simulink model "Fusion_Frame_Model_Architecture"  (R2018a)
settings: Solver=FixedStepAuto  StartTime=0.0  StopTime=SimulationTime  FixedStep=SamplingTime  RelTol=1e-3
undefined symbols (not defined in the file or in its folder): ACTIVATE_CAM, ACTIVATE_RAD, CAM1_detTimeStamp, CAM1_MeasNoise, CAM1_objClassID, CAM1_PX, CAM1_PY, CAM1_VX, CAM1_VY, CAM2_detTimeStamp, CAM2_MeasNoise, CAM2_objClassID, CAM2_PX, CAM2_PY, CAM2_VX, CAM2_VY, CAM3_detTimeStamp, CAM3_MeasNoise, CAM3_objClassID, CAM3_PX, CAM3_PY, CAM3_VX, CAM3_VY, CAM4_detTimeStamp, CAM4_MeasNoise, CAM4_objClassID, CAM4_PX, CAM4_PY, CAM4_VX, CAM4_VY, CAM5_detTimeStamp, CAM5_MeasNoise, CAM5_objClassID, CAM5_PX, CAM5_PY, CAM5_VX, CAM5_VY, CAM6_detTimeStamp, CAM6_MeasNoise, CAM6_objClassID, CAM6_PX, CAM6_PY, CAM6_VX, CAM6_VY, CAM7_detTimeStamp, CAM7_MeasNoise, CAM7_objClassID, CAM7_PX, CAM7_PY, CAM7_VX, CAM7_VY, CAM8_detTimeStamp, CAM8_MeasNoise, CAM8_objClassID, CAM8_PX, CAM8_PY, CAM8_VX, CAM8_VY, CAM_nMeas, CAM_TYPE ... (+181)
libraries: simulink_extras x4
(part 2 of 11)

== system Fusion_Frame_Model_Architecture/SENSOR_FUSION_SYSTEM/OBJECT_TRACKER_SENSOR_FUSION/RADAR_HOMOGENEOUS_FUSION/GATING ==
  MEAS : Inport
  RAD_PARAM : Inport  Port=2
  RADAR_CLUSTERS : Inport  Port=3
  TrackParamPred : Inport  Port=4
  FIND_UNASSOCIATED_CLUSTERS : Subsystem
  GET_DATA : Subsystem
  MEASUREMENT_TO_TRACK_GATING_AND_LOGLIKELIHOOD_COMPUTATION : Subsystem
  RESOLVE_GATING_AMBIGUITY : Subsystem
  GatedMeasFlag : Outport
  GatedMeasLogLikelihood : Outport  Port=2
  UnGatedMeasCluster : Outport  Port=3
  wires:
  MEAS/1 -> MEASUREMENT_TO_TRACK_GATING_AND_LOGLIKELIHOOD_COMPUTATION/4(Meas), FIND_UNASSOCIATED_CLUSTERS/3(measCLUSTERS)
  MEASUREMENT_TO_TRACK_GATING_AND_LOGLIKELIHOOD_COMPUTATION/2(GatedMeasFlagArray) -> RESOLVE_GATING_AMBIGUITY/3(GatedMeasFlagArrayIn)
  MEASUREMENT_TO_TRACK_GATING_AND_LOGLIKELIHOOD_COMPUTATION/3(GatedMeasLogLikelihood) -> RESOLVE_GATING_AMBIGUITY/4(GatedMeasLogLikelihoodIn)
  TrackParamPred/1 -> GET_DATA/1(TRACKS)
  GET_DATA/1(nTracksPred) -> MEASUREMENT_TO_TRACK_GATING_AND_LOGLIKELIHOOD_COMPUTATION/1(nTracks), RESOLVE_GATING_AMBIGUITY/1(nTracks)
  GET_DATA/2(TrackParam) -> MEASUREMENT_TO_TRACK_GATING_AND_LOGLIKELIHOOD_COMPUTATION/2(TrackParamPred)
  MEASUREMENT_TO_TRACK_GATING_AND_LOGLIKELIHOOD_COMPUTATION/1(nMeas) -> RESOLVE_GATING_AMBIGUITY/2(nMeas)
  RESOLVE_GATING_AMBIGUITY/1(GatedMeasFlagArray) -> GatedMeasFlag/1, FIND_UNASSOCIATED_CLUSTERS/1(GatedMeasFlagArray)
  RADAR_CLUSTERS/1 -> FIND_UNASSOCIATED_CLUSTERS/2(Clusters)
  RESOLVE_GATING_AMBIGUITY/2(GatedMeasLogLikelihood) -> GatedMeasLogLikelihood/1
  FIND_UNASSOCIATED_CLUSTERS/1(UngatedCLUSTERS) -> UnGatedMeasCluster/1
  RAD_PARAM/1 -> MEASUREMENT_TO_TRACK_GATING_AND_LOGLIKELIHOOD_COMPUTATION/3(SnsrParam)

== system Fusion_Frame_Model_Architecture/SENSOR_FUSION_SYSTEM/OBJECT_TRACKER_SENSOR_FUSION/RADAR_HOMOGENEOUS_FUSION/SEGREGATE_CLUSTER ==
  RADAR_MEAS : Inport
  RADAR_CLUSTERS : Inport  Port=2
  Bus Creator : BusCreator  Inputs=5  OutDataTypeStr=Bus: RAD_MEAS_MAT_CTS  NonVirtualBus=on
      settings: InheritFromInputs=off
  MATLAB Function : MATLAB Function  TreatAsAtomicUnit=on
  Spatially_Alligned_Snsr_Meas_Plots : Subsystem
  RADAR_CLSTR_MEAS : Outport
  wires:
  RADAR_MEAS/1 -> MATLAB Function/1(SENSORMeasCTS)
  RADAR_CLUSTERS/1 -> MATLAB Function/2(SENSOR_CLUSTERS)
  Bus Creator/1 -> Spatially_Alligned_Snsr_Meas_Plots/1(RAD_MEAS), RADAR_CLSTR_MEAS/1
  MATLAB Function/1(MeasArray) -> Bus Creator/1  "MeasArray"
  MATLAB Function/2(MeasCovariance) -> Bus Creator/2  "MeasCovariance"
  MATLAB Function/3(ClusterRef) -> Bus Creator/3  "MeasRef"
  MATLAB Function/4(ValidMeasCount) -> Bus Creator/4  "ValidMeasCount"
  MATLAB Function/5(ValidCumulativeMeasCount) -> Bus Creator/5  "ValidCumulativeMeasCount"

== system Fusion_Frame_Model_Architecture/SENSOR_FUSION_SYSTEM/OBJECT_TRACKER_SENSOR_FUSION/RADAR_HOMOGENEOUS_FUSION/SIMPLYFIED_DBSCAN_FOR_RADAR_MEASUREMENT_GROUPING ==
  RADAR_MEAS : Inport
  DBSCAN_MEASUREMENT_GROUPING : Subsystem  TreatAsAtomicUnit=on
  GET_NUM_OF_MEAS : Subsystem
  RADAR_CLUSTERS : Outport
  wires:
  GET_NUM_OF_MEAS/1(nMeas) -> DBSCAN_MEASUREMENT_GROUPING/1(nMeas)
  RADAR_MEAS/1 -> GET_NUM_OF_MEAS/1(RAD_MEAS_CTS), DBSCAN_MEASUREMENT_GROUPING/2(Meas)
  DBSCAN_MEASUREMENT_GROUPING/1(RADAR_CLUSTERS) -> RADAR_CLUSTERS/1

== system Fusion_Frame_Model_Architecture/SENSOR_FUSION_SYSTEM/OBJECT_TRACKER_SENSOR_FUSION/RADAR_HOMOGENEOUS_FUSION/STATE_PREDICTION ==
  TrackParamPrev : Inport
  GET_DATA : Subsystem
  SET_DATA : Subsystem
  TRACK_STATE_PREDICTION : Subsystem
  Unit Delay : UnitDelay  InitialCondition=TRACK_EST_RAD_INIT  SampleTime=-1
  TrackParamPred : Outport
  wires:
  TrackParamPrev/1 -> Unit Delay/1
  Unit Delay/1 -> GET_DATA/1(TRACKS), SET_DATA/1(TRACKS_in)
  GET_DATA/1(nTracksPrev) -> TRACK_STATE_PREDICTION/1(nTracks)
  GET_DATA/2(TrackParam) -> TRACK_STATE_PREDICTION/2(TrackParamPred)
  TRACK_STATE_PREDICTION/1(StatePredBus) -> SET_DATA/2(TrackParam)
  SET_DATA/1(TRACKS) -> TrackParamPred/1

== system Fusion_Frame_Model_Architecture/SENSOR_FUSION_SYSTEM/OBJECT_TRACKER_SENSOR_FUSION/RADAR_HOMOGENEOUS_FUSION/TRACK_MANAGER ==
  TrackParamIn : Inport
  UnGatedClusters : Inport  Port=2
  Grid : Inport  Port=3
  Bus Creator : BusCreator  Inputs=6  OutDataTypeStr=Bus: TRACK_ESTIMATES_BUS  NonVirtualBus=on
      settings: InheritFromInputs=off
  Bus Selector : BusSelector  OutputSignals=nValidTracks,TrackParam,TrackIDList,IsTrackIDused,FirstAvailableIDindex,LastAvailableIDindex
  Terminator : Terminator
  Terminator1 : Terminator
  TrackParamUpd : Outport
  wires:
  UnGatedClusters/1 -> Terminator/1
  Bus Creator/1 -> TrackParamUpd/1
  Bus Selector/4 -> Bus Creator/4  "<IsTrackIDused>"
  Bus Selector/2 -> Bus Creator/2  "<TrackParam>"
  Bus Selector/3 -> Bus Creator/3  "<TrackIDList>"
  TrackParamIn/1 -> Bus Selector/1
  Bus Selector/1 -> Bus Creator/1  "<nValidTracks>"
  Bus Selector/5 -> Bus Creator/5  "<FirstAvailableIDindex>"
  Bus Selector/6 -> Bus Creator/6  "<LastAvailableIDindex>"
  Grid/1 -> Terminator1/1

== system Fusion_Frame_Model_Architecture/SENSOR_FUSION_SYSTEM/OBJECT_TRACKER_SENSOR_FUSION/SENSOR_LAYOUT_AND_CHRACTERIZATION/PRE_COMPUTE_SENSOR_FOV_GRID ==
  RADSnsrParam : Inport
  CAMSnsrParam : Inport  Port=2
  COMPUTE_CAMERA_SNSR_GRID : Subsystem
  COMPUTE_GRID_DIMENSION : Subsystem
  COMPUTE_RADAR_SNSR_GRID : Subsystem
  CREATE_GRID : Subsystem  TreatAsAtomicUnit=on
  SET_DATA : Subsystem
  GRID_CHARACTERIZATION : Outport
  wires:
  RADSnsrParam/1 -> COMPUTE_RADAR_SNSR_GRID/1(SnsrParam)
  COMPUTE_GRID_DIMENSION/2(Cy) -> CREATE_GRID/2(Cy)
  COMPUTE_GRID_DIMENSION/3(GridParam) -> [GridParam], CREATE_GRID/3(GridParam)
  COMPUTE_GRID_DIMENSION/1(Cx) -> CREATE_GRID/1(Cx)
  CREATE_GRID/1(CellIDVectorUpd) -> COMPUTE_CAMERA_SNSR_GRID/1(GridIDVector), COMPUTE_RADAR_SNSR_GRID/3(GridIDVector)
  [GridParam] -> COMPUTE_RADAR_SNSR_GRID/2(GridParam)
  [GridParam] -> COMPUTE_CAMERA_SNSR_GRID/2(GridParam)
  CAMSnsrParam/1 -> COMPUTE_CAMERA_SNSR_GRID/3(SnsrParam)
  [GridParam] -> SET_DATA/1(GRID_PARAM)  "GRID_PARAM"
  COMPUTE_RADAR_SNSR_GRID/1(RegionConfidence) -> SET_DATA/2(RAD_REGION_CONFIDENCE)  "RAD_REGION_CONFIDENCE"
  COMPUTE_RADAR_SNSR_GRID/2(FOVOverlap) -> SET_DATA/3(RAD_FOV_OVERLAP)  "RAD_FOV_OVERLAP"
  COMPUTE_CAMERA_SNSR_GRID/1(RegionConfidence) -> SET_DATA/4(CAM_REGION_CONFIDENCE)  "CAM_REGION_CONFIDENCE"
  COMPUTE_CAMERA_SNSR_GRID/2(FOVOverlap) -> SET_DATA/5(CAM_FOV_OVERLAP)  "CAM_FOV_OVERLAP"
  SET_DATA/1(GRID_CHARACTERIZATION) -> GRID_CHARACTERIZATION/1

== system Fusion_Frame_Model_Architecture/SENSOR_FUSION_SYSTEM/OBJECT_TRACKER_SENSOR_FUSION/SENSOR_LAYOUT_AND_CHRACTERIZATION/SET_SENSOR_CALLIBRATION_PARAMETER ==
  CamCalibParam : Inport  OutDataTypeStr=Bus: CAM_SENSOR_PARAM  PortDimensions=nCameraActive  BusOutputAsStruct=on
  RADSnsrParam : Inport  Port=2  OutDataTypeStr=Bus: RAD_SENSOR_PARAM  PortDimensions=1
  SET_CAMERA_SENSOR_PARAM : Subsystem  TreatAsAtomicUnit=on
  SET_RADAR_SENSOR_PARAM : Subsystem
  RadarCalibParamUpd : Outport
  CameraCalibParamUpd : Outport  Port=2
  wires:
  SET_CAMERA_SENSOR_PARAM/1(CAMSnsrParamUpd) -> CameraCalibParamUpd/1
  CamCalibParam/1 -> SET_CAMERA_SENSOR_PARAM/1(CAMSnsrParam)
  RADSnsrParam/1 -> SET_RADAR_SENSOR_PARAM/1(RADSnsrParam)
  SET_RADAR_SENSOR_PARAM/1(RADSnsrParamUpd) -> RadarCalibParamUpd/1

== system Fusion_Frame_Model_Architecture/SENSOR_FUSION_SYSTEM/OBJECT_TRACKER_SENSOR_FUSION/SPATIAL_ALLIGNMENT1/CAMERA_MEASUREMENTS_SPATIAL_ALLIGNMENT ==
  CameraCalibParam : Inport  BusOutputAsStruct=on
  C1 : Inport  Port=2
  C2 : Inport  Port=3
  C3 : Inport  Port=4
  C4 : Inport  Port=5
  C5 : Inport  Port=6
  C6 : Inport  Port=7
  C7 : Inport  Port=8
  C8 : Inport  Port=9
  For Iterator Subsystem : Subsystem  TreatAsAtomicUnit=on
  RadarMeasurementIndexes2 : Subsystem
  StartingIndexes1 : Subsystem
  CameraMeasTransformed : Outport
  wires:
  CameraCalibParam/1 -> For Iterator Subsystem/1(CameraCallibrationParam), StartingIndexes1/1(SnsrCallib)
  C6/1 -> For Iterator Subsystem/8(C6)
  C3/1 -> For Iterator Subsystem/5(C3)
  C4/1 -> For Iterator Subsystem/6(C4)
  C2/1 -> For Iterator Subsystem/4(C2)
  C1/1 -> For Iterator Subsystem/3(C1)
  StartingIndexes1/1(StartingIndexes) -> For Iterator Subsystem/2(RadarStartingIdx)
  C5/1 -> For Iterator Subsystem/7(C5)
  C7/1 -> For Iterator Subsystem/9(C7)
  C8/1 -> For Iterator Subsystem/10(C8)
  For Iterator Subsystem/2(CameraMeasTransformed) -> RadarMeasurementIndexes2/2(CTSmeasMAT)
  RadarMeasurementIndexes2/1(CTSmeasMATout) -> CameraMeasTransformed/1
  For Iterator Subsystem/4(CameraMeasRef) -> RadarMeasurementIndexes2/4(CTSRefMAT)
  For Iterator Subsystem/3(CameraMeasCOVTransformed) -> RadarMeasurementIndexes2/3(CTSCovMAT)
  For Iterator Subsystem/1(MaxNoValidMeas) -> RadarMeasurementIndexes2/1(validMeasCount)

== system Fusion_Frame_Model_Architecture/SENSOR_FUSION_SYSTEM/OBJECT_TRACKER_SENSOR_FUSION/SPATIAL_ALLIGNMENT1/GET_CAM_MEAS ==
  CameraParam : Inport
  CameraMeas : Inport  Port=2
  Bus Selector1 : BusSelector  OutputSignals=C1,C2,C3,C4,C5,C6,C7,C8
  Bus Selector2 : BusSelector  OutputSignals=CameraExtrinsics
  SnsrParam : Outport
  <C1> : Outport  Port=2
  <C2> : Outport  Port=3
  <C3> : Outport  Port=4
  <C4> : Outport  Port=5
  <C5> : Outport  Port=6
  <C6> : Outport  Port=7
  <C7> : Outport  Port=8
  <C8> : Outport  Port=9
  wires:
  Bus Selector1/4 -> <C4>/1  "<C4>"
  Bus Selector1/6 -> <C6>/1  "<C6>"
  Bus Selector1/5 -> <C5>/1  "<C5>"
  CameraMeas/1 -> Bus Selector1/1
  Bus Selector1/1 -> <C1>/1  "<C1>"
  Bus Selector1/7 -> <C7>/1  "<C7>"
  Bus Selector1/8 -> <C8>/1  "<C8>"
  Bus Selector1/2 -> <C2>/1  "<C2>"
  Bus Selector1/3 -> <C3>/1  "<C3>"
  CameraParam/1 -> Bus Selector2/1
  Bus Selector2/1 -> SnsrParam/1  "<CameraExtrinsics>"

== system Fusion_Frame_Model_Architecture/SENSOR_FUSION_SYSTEM/OBJECT_TRACKER_SENSOR_FUSION/SPATIAL_ALLIGNMENT1/GET_RAD_MEAS ==
  RadarParam : Inport
  RadarMeas : Inport  Port=2
  Bus Selector : BusSelector  OutputSignals=R1,R2,R3,R4,R5,R6
  Bus Selector1 : BusSelector  OutputSignals=RadarExtrinsics
  SnsrParam : Outport
  <R1> : Outport  Port=2
  <R2> : Outport  Port=3
  <R3> : Outport  Port=4
  <R4> : Outport  Port=5
  <R5> : Outport  Port=6
  <R6> : Outport  Port=7
  wires:
  Bus Selector/1 -> <R1>/1  "<R1>"
  Bus Selector/2 -> <R2>/1  "<R2>"
  Bus Selector/3 -> <R3>/1  "<R3>"
  Bus Selector/6 -> <R6>/1  "<R6>"
  Bus Selector/4 -> <R4>/1  "<R4>"
  Bus Selector/5 -> <R5>/1  "<R5>"
  RadarMeas/1 -> Bus Selector/1
  Bus Selector1/1 -> SnsrParam/1  "<RadarExtrinsics>"
  RadarParam/1 -> Bus Selector1/1

== system Fusion_Frame_Model_Architecture/SENSOR_FUSION_SYSTEM/OBJECT_TRACKER_SENSOR_FUSION/SPATIAL_ALLIGNMENT1/RADAR_MEASUREMENTS_SPATIAL_ALLIGNMENT ==
  RadarCalibParam : Inport  BusOutputAsStruct=on
  R1 : Inport  Port=2
  R2 : Inport  Port=3
  R3 : Inport  Port=4
  R4 : Inport  Port=5
  R5 : Inport  Port=6
  R6 : Inport  Port=7
  RADAR_MEASUREMENTS_SPATIAL_ALLIGNMENT : Subsystem  TreatAsAtomicUnit=on
  SET_MEASUREMENTS : Subsystem
  StartingIndexes1 : Subsystem
  RadarMeasTransformed : Outport
  wires:
  StartingIndexes1/1(StartingIndexes) -> RADAR_MEASUREMENTS_SPATIAL_ALLIGNMENT/2(RadarStartingIdx)
  R1/1 -> RADAR_MEASUREMENTS_SPATIAL_ALLIGNMENT/3(R1)
  R2/1 -> RADAR_MEASUREMENTS_SPATIAL_ALLIGNMENT/4(R2)
  R4/1 -> RADAR_MEASUREMENTS_SPATIAL_ALLIGNMENT/6(R4)
  R5/1 -> RADAR_MEASUREMENTS_SPATIAL_ALLIGNMENT/7(R5)
  RadarCalibParam/1 -> RADAR_MEASUREMENTS_SPATIAL_ALLIGNMENT/1(RadarCallibrationParam), StartingIndexes1/1(SnsrCallib)
  R6/1 -> RADAR_MEASUREMENTS_SPATIAL_ALLIGNMENT/8(R6)
  R3/1 -> RADAR_MEASUREMENTS_SPATIAL_ALLIGNMENT/5(R3)
  RADAR_MEASUREMENTS_SPATIAL_ALLIGNMENT/1(RadarMeasTransformed) -> SET_MEASUREMENTS/1(CTSmeasMAT)
  RADAR_MEASUREMENTS_SPATIAL_ALLIGNMENT/4(MaxNoValidMeas) -> SET_MEASUREMENTS/4(validMeasCount)
  SET_MEASUREMENTS/1(CTSmeasMATout) -> RadarMeasTransformed/1
  RADAR_MEASUREMENTS_SPATIAL_ALLIGNMENT/2(RadarMeasCOVTransformed) -> SET_MEASUREMENTS/2(CTSCovMAT)
  RADAR_MEASUREMENTS_SPATIAL_ALLIGNMENT/3(RadarMeasRef) -> SET_MEASUREMENTS/3(CTSRefMAT)

== system Fusion_Frame_Model_Architecture/SENSOR_FUSION_SYSTEM/OBJECT_TRACKER_SENSOR_FUSION/TRACKS_TRAJECTORY_COMPUTATION/EGO_COMPENSATE_TRAJECTORY_HISTORY_BUFFER ==
  RAD_CAM_TRACKS_FUS : Inport
  TRAJECTORIES : Inport  Port=2
  Bus Creator : BusCreator  Inputs=2  OutDataTypeStr=Bus: TRAJECTORY_HISTORY_BUS  NonVirtualBus=on
      settings: InheritFromInputs=off
  Bus Selector : BusSelector  OutputSignals=nConfirmedTracks,TrackHistory
  Terminator : Terminator
  TRAJECTORIES_UPD : Outport
  wires:
  RAD_CAM_TRACKS_FUS/1 -> Terminator/1
  Bus Selector/2 -> Bus Creator/2  "<TrackHistory>"
  Bus Selector/1 -> Bus Creator/1  "<nConfirmedTracks>"
  TRAJECTORIES/1 -> Bus Selector/1
  Bus Creator/1 -> TRAJECTORIES_UPD/1

== system Fusion_Frame_Model_Architecture/SENSOR_FUSION_SYSTEM/OBJECT_TRACKER_SENSOR_FUSION/TRACKS_TRAJECTORY_COMPUTATION/UPDATE_TRAJECTORY_BUFFER_WITH_CURRENT_TRACK_DATA ==
  RAD_CAM_TRACKS_FUS : Inport
  TRAJECTORIES : Inport  Port=2
  Terminator : Terminator
  Unit Delay : UnitDelay  InitialCondition=TRACK_HISTORY_INIT  SampleTime=-1
  TRAJECTORIES_UPD : Outport
  wires:
  TRAJECTORIES/1 -> Unit Delay/1
  Unit Delay/1 -> TRAJECTORIES_UPD/1
  RAD_CAM_TRACKS_FUS/1 -> Terminator/1

== system Fusion_Frame_Model_Architecture/SENSOR_FUSION_SYSTEM/ROAD_GEOMETRY_CAMERA_FUSION/EGO_LANE_CENTER_LINE_ESTIMATION_FROM_LEFT_BOUNDARY/CURVE_FITTING_BY_LEAST_SQUARES ==
  Points : Inport
  Ground : Ground
  Terminator : Terminator
  PolynomialCoefficients : Outport
  wires:
  Points/1 -> Terminator/1
  Ground/1 -> PolynomialCoefficients/1

== system Fusion_Frame_Model_Architecture/SENSOR_FUSION_SYSTEM/ROAD_GEOMETRY_CAMERA_FUSION/EGO_LANE_CENTER_LINE_ESTIMATION_FROM_LEFT_BOUNDARY/GENERATE_POINTS_AT_EGO_LANE_CENTER ==
  PointsAlongTheLine : Inport
  EgoLaneWidth : Inport  Port=2
  Ground : Ground
  Terminator : Terminator
  Terminator1 : Terminator
  PointsAlongEgoLaneCenter : Outport
  wires:
  PointsAlongTheLine/1 -> Terminator/1
  Ground/1 -> PointsAlongEgoLaneCenter/1
  EgoLaneWidth/1 -> Terminator1/1

== system Fusion_Frame_Model_Architecture/SENSOR_FUSION_SYSTEM/ROAD_GEOMETRY_CAMERA_FUSION/EGO_LANE_CENTER_LINE_ESTIMATION_FROM_LEFT_BOUNDARY/INTERPOLATE_POINTS_ALONG_THE_LINE ==
  LEFT_LINE_TRACK : Inport
  Ground : Ground
  Terminator : Terminator
  PointsAlongTheLine : Outport
  wires:
  LEFT_LINE_TRACK/1 -> Terminator/1
  Ground/1 -> PointsAlongTheLine/1

== system Fusion_Frame_Model_Architecture/SENSOR_FUSION_SYSTEM/ROAD_GEOMETRY_CAMERA_FUSION/EGO_LANE_CENTER_LINE_ESTIMATION_FROM_LEFT_BOUNDARY/KALMAN_FILTER_STATE_UPDATE ==
  CenterLineHypothesis : Inport
  CenterLinePred : Inport  Port=2
  Terminator : Terminator
  Unit Delay : UnitDelay  InitialCondition=LANE_LINE_TRACK  SampleTime=-1
  CenterLineHypUpd : Outport
  wires:
  CenterLineHypothesis/1 -> Terminator/1
  CenterLinePred/1 -> Unit Delay/1
  Unit Delay/1 -> CenterLineHypUpd/1

== system Fusion_Frame_Model_Architecture/SENSOR_FUSION_SYSTEM/ROAD_GEOMETRY_CAMERA_FUSION/EGO_LANE_CENTER_LINE_ESTIMATION_FROM_LEFT_BOUNDARY/POLYNOMIAL_TO_CLOTHOID_CONVERSION ==
  PolynomialCoefficients : Inport
  Ground : Ground
  Terminator : Terminator
  ClothoidCoefficients : Outport
  wires:
  PolynomialCoefficients/1 -> Terminator/1
  Ground/1 -> ClothoidCoefficients/1

== system Fusion_Frame_Model_Architecture/SENSOR_FUSION_SYSTEM/ROAD_GEOMETRY_CAMERA_FUSION/EGO_LANE_CENTER_LINE_ESTIMATION_FROM_RIGHT_BOUNDARY/CURVE_FITTING_BY_LEAST_SQUARES ==
  Points : Inport
  Ground : Ground
  Terminator : Terminator
  PolynomialCoefficients : Outport
  wires:
  Points/1 -> Terminator/1
  Ground/1 -> PolynomialCoefficients/1

== system Fusion_Frame_Model_Architecture/SENSOR_FUSION_SYSTEM/ROAD_GEOMETRY_CAMERA_FUSION/EGO_LANE_CENTER_LINE_ESTIMATION_FROM_RIGHT_BOUNDARY/GENERATE_POINTS_AT_EGO_LANE_CENTER ==
  PointsAlongTheLine : Inport
  EgoLaneWidth : Inport  Port=2
  Ground : Ground
  Terminator : Terminator
  Terminator1 : Terminator
  PointsAlongEgoLaneCenter : Outport
  wires:
  PointsAlongTheLine/1 -> Terminator/1
  Ground/1 -> PointsAlongEgoLaneCenter/1
  EgoLaneWidth/1 -> Terminator1/1

== system Fusion_Frame_Model_Architecture/SENSOR_FUSION_SYSTEM/ROAD_GEOMETRY_CAMERA_FUSION/EGO_LANE_CENTER_LINE_ESTIMATION_FROM_RIGHT_BOUNDARY/INTERPOLATE_POINTS_ALONG_THE_LINE ==
  LEFT_LINE_TRACK : Inport
  Ground : Ground
  Terminator : Terminator
  PointsAlongTheLine : Outport
  wires:
  LEFT_LINE_TRACK/1 -> Terminator/1
  Ground/1 -> PointsAlongTheLine/1

== system Fusion_Frame_Model_Architecture/SENSOR_FUSION_SYSTEM/ROAD_GEOMETRY_CAMERA_FUSION/EGO_LANE_CENTER_LINE_ESTIMATION_FROM_RIGHT_BOUNDARY/KALMAN_FILTER_STATE_UPDATE ==
  CenterLineHypothesis : Inport
  CenterLinePred : Inport  Port=2
  Terminator : Terminator
  Unit Delay : UnitDelay  InitialCondition=LANE_LINE_TRACK  SampleTime=-1
  CenterLineHypUpd : Outport
  wires:
  CenterLineHypothesis/1 -> Terminator/1
  CenterLinePred/1 -> Unit Delay/1
  Unit Delay/1 -> CenterLineHypUpd/1

== system Fusion_Frame_Model_Architecture/SENSOR_FUSION_SYSTEM/ROAD_GEOMETRY_CAMERA_FUSION/EGO_LANE_CENTER_LINE_ESTIMATION_FROM_RIGHT_BOUNDARY/POLYNOMIAL_TO_CLOTHOID_CONVERSION ==
  PolynomialCoefficients : Inport
  Ground : Ground
  Terminator : Terminator
  ClothoidCoefficients : Outport
  wires:
  PolynomialCoefficients/1 -> Terminator/1
  Ground/1 -> ClothoidCoefficients/1

== system Fusion_Frame_Model_Architecture/SENSOR_FUSION_SYSTEM/ROAD_GEOMETRY_CAMERA_FUSION/EGO_LANE_CENTER_LINE_HYPOTHESIS_FUSION/EGO_LANE_CENTER_LINE_PREDICTION ==
  EGO_LANE_CENTER_LINE : Inport
  Bus Creator : BusCreator  Inputs=7  OutDataTypeStr=Bus: ClothoidParamBus  NonVirtualBus=on
      settings: InheritFromInputs=off
  Bus Selector : BusSelector  OutputSignals=LateralOffset,HeadingAngle,Curvature,CurvatureDerivative,CurveLengthStart,CurveLength,ErrCOV
  EGO_LANE_CENTER_LINE_PRED : Outport
  wires:
  Bus Creator/1 -> EGO_LANE_CENTER_LINE_PRED/1
  Bus Selector/6 -> Bus Creator/6  "<CurveLength>"
  Bus Selector/5 -> Bus Creator/5  "<CurveLengthStart>"
  Bus Selector/4 -> Bus Creator/4  "<CurvatureDerivative>"
  Bus Selector/1 -> Bus Creator/1  "<LateralOffset>"
  Bus Selector/3 -> Bus Creator/3  "<Curvature>"
  EGO_LANE_CENTER_LINE/1 -> Bus Selector/1
  Bus Selector/2 -> Bus Creator/2  "<HeadingAngle>"
  Bus Selector/7 -> Bus Creator/7  "<ErrCOV>"

== system Fusion_Frame_Model_Architecture/SENSOR_FUSION_SYSTEM/ROAD_GEOMETRY_CAMERA_FUSION/EGO_LANE_CENTER_LINE_HYPOTHESIS_FUSION/HYPOTHESIS_MERGE ==
  EGO_LANE_CENTER_LINE_HYP1 : Inport
  weight : Inport  Port=2
  EGO_LANE_CENTER_LINE_HYP2 : Inport  Port=3
  Terminator1 : Terminator
  Terminator2 : Terminator
  EGO_LANE_CENTER_LINE : Outport
  wires:
  EGO_LANE_CENTER_LINE_HYP1/1 -> EGO_LANE_CENTER_LINE/1
  EGO_LANE_CENTER_LINE_HYP2/1 -> Terminator1/1
  weight/1 -> Terminator2/1

== system Fusion_Frame_Model_Architecture/SENSOR_FUSION_SYSTEM/ROAD_GEOMETRY_CAMERA_FUSION/EGO_LANE_CENTER_LINE_HYPOTHESIS_FUSION/WEIGHTAGE_COMPUTATION ==
  EGO_LANE_CENTER_LINE_HYP1 : Inport
  EGO_LANE_CENTER_LINE_HYP2 : Inport  Port=2
  Ground : Ground
  Terminator : Terminator
  Terminator1 : Terminator
  weight : Outport
  wires:
  EGO_LANE_CENTER_LINE_HYP1/1 -> Terminator/1
  EGO_LANE_CENTER_LINE_HYP2/1 -> Terminator1/1
  Ground/1 -> weight/1

== system Fusion_Frame_Model_Architecture/SENSOR_FUSION_SYSTEM/ROAD_GEOMETRY_CAMERA_FUSION/EGO_LANE_LEFT_BOUNDARY_LINE_FUSION/FIND_UNGATED_LINE_MEASUREMENTS ==
  GatedMeasIndex : Inport
  EGO_LANE_LEFT_LINE_MEAS : Inport  Port=2
  Ground : Ground
  Terminator1 : Terminator
  Terminator2 : Terminator
  UnGatedMeasIndex : Outport
  wires:
  EGO_LANE_LEFT_LINE_MEAS/1 -> Terminator1/1
  GatedMeasIndex/1 -> Terminator2/1
  Ground/1 -> UnGatedMeasIndex/1

== system Fusion_Frame_Model_Architecture/SENSOR_FUSION_SYSTEM/ROAD_GEOMETRY_CAMERA_FUSION/EGO_LANE_LEFT_BOUNDARY_LINE_FUSION/LANE_LINE_MEASUREMENT_TO_TRACK_FUSION ==
  GatedMeasIndex : Inport
  TrackParamPred : Inport  Port=2
  EGO_LANE_LEFT_LINE_MEAS : Inport  Port=3
  Terminator1 : Terminator
  Terminator2 : Terminator
  TrackParamUpd : Outport
  wires:
  TrackParamPred/1 -> TrackParamUpd/1
  EGO_LANE_LEFT_LINE_MEAS/1 -> Terminator1/1
  GatedMeasIndex/1 -> Terminator2/1

== system Fusion_Frame_Model_Architecture/SENSOR_FUSION_SYSTEM/ROAD_GEOMETRY_CAMERA_FUSION/EGO_LANE_LEFT_BOUNDARY_LINE_FUSION/LANE_LINE_MEASUREMENT_TO_TRACK_GATING ==
  TrackParamPred : Inport
  EGO_LANE_LEFT_LINE_MEAS : Inport  Port=2
  Ground : Ground
  Terminator : Terminator
  Terminator1 : Terminator
  GatedMeasIndex : Outport
  wires:
  TrackParamPred/1 -> Terminator/1
  Ground/1 -> GatedMeasIndex/1
  EGO_LANE_LEFT_LINE_MEAS/1 -> Terminator1/1

== system Fusion_Frame_Model_Architecture/SENSOR_FUSION_SYSTEM/ROAD_GEOMETRY_CAMERA_FUSION/EGO_LANE_LEFT_BOUNDARY_LINE_FUSION/LANE_LINE_STATE_PREDICTION ==
  TrackParamPrev : Inport
  Unit Delay : UnitDelay  InitialCondition=LANE_LINE_TRACK  SampleTime=-1
  TrackParamPred : Outport
  wires:
  TrackParamPrev/1 -> Unit Delay/1
  Unit Delay/1 -> TrackParamPred/1

== system Fusion_Frame_Model_Architecture/SENSOR_FUSION_SYSTEM/ROAD_GEOMETRY_CAMERA_FUSION/EGO_LANE_LEFT_BOUNDARY_LINE_FUSION/LINE_TRACK_MANAGER ==
  UnGatedMeasIndex : Inport
  TrackParamUpd_in : Inport  Port=2
  Line_Measurements : Inport  Port=3
  Bus Creator : BusCreator  Inputs=7  OutDataTypeStr=Bus: ClothoidParamBus  NonVirtualBus=on
      settings: InheritFromInputs=off
  Bus Selector : BusSelector  OutputSignals=LateralOffset,HeadingAngle,Curvature,CurvatureDerivative,CurveLengthStart,CurveLength,ErrCOV
  Terminator : Terminator
  Terminator1 : Terminator
  TrackParamUpd : Outport
  wires:
  UnGatedMeasIndex/1 -> Terminator/1
  Line_Measurements/1 -> Terminator1/1
  Bus Selector/7 -> Bus Creator/7  "<ErrCOV>"
  Bus Selector/3 -> Bus Creator/3  "<Curvature>"
  Bus Creator/1 -> TrackParamUpd/1
  Bus Selector/4 -> Bus Creator/4  "<CurvatureDerivative>"
  Bus Selector/6 -> Bus Creator/6  "<CurveLength>"
  Bus Selector/1 -> Bus Creator/1  "<LateralOffset>"
  Bus Selector/2 -> Bus Creator/2  "<HeadingAngle>"
  Bus Selector/5 -> Bus Creator/5  "<CurveLengthStart>"
  TrackParamUpd_in/1 -> Bus Selector/1

== system Fusion_Frame_Model_Architecture/SENSOR_FUSION_SYSTEM/ROAD_GEOMETRY_CAMERA_FUSION/EGO_LANE_RIGHT_BOUNDARY_LINE_FUSION/FIND_UNGATED_LINE_MEASUREMENTS ==
  GatedMeasIndex : Inport
  EGO_LANE_RIGHT_LINE_MEAS : Inport  Port=2
  Ground : Ground
  Terminator1 : Terminator
  Terminator2 : Terminator
  UnGatedMeasIndex : Outport
  wires:
  EGO_LANE_RIGHT_LINE_MEAS/1 -> Terminator1/1
  GatedMeasIndex/1 -> Terminator2/1
  Ground/1 -> UnGatedMeasIndex/1

== system Fusion_Frame_Model_Architecture/SENSOR_FUSION_SYSTEM/ROAD_GEOMETRY_CAMERA_FUSION/EGO_LANE_RIGHT_BOUNDARY_LINE_FUSION/LANE_LINE_MEASUREMENT_TO_TRACK_FUSION ==
  GatedMeasIndex : Inport
  TrackParamPred : Inport  Port=2
  EGO_LANE_RIGHT_LINE_MEAS : Inport  Port=3
  Terminator1 : Terminator
  Terminator2 : Terminator
  TrackParamUpd : Outport
  wires:
  TrackParamPred/1 -> TrackParamUpd/1
  EGO_LANE_RIGHT_LINE_MEAS/1 -> Terminator1/1
  GatedMeasIndex/1 -> Terminator2/1

== system Fusion_Frame_Model_Architecture/SENSOR_FUSION_SYSTEM/ROAD_GEOMETRY_CAMERA_FUSION/EGO_LANE_RIGHT_BOUNDARY_LINE_FUSION/LANE_LINE_MEASUREMENT_TO_TRACK_GATING ==
  TrackParamPred : Inport
  EGO_LANE_RIGHT_LINE_MEAS : Inport  Port=2
  Ground : Ground
  Terminator : Terminator
  Terminator1 : Terminator
  GatedMeasIndex : Outport
  wires:
  TrackParamPred/1 -> Terminator/1
  Ground/1 -> GatedMeasIndex/1
  EGO_LANE_RIGHT_LINE_MEAS/1 -> Terminator1/1

== system Fusion_Frame_Model_Architecture/SENSOR_FUSION_SYSTEM/ROAD_GEOMETRY_CAMERA_FUSION/EGO_LANE_RIGHT_BOUNDARY_LINE_FUSION/LANE_LINE_STATE_PREDICTION ==
  TrackParamPrev : Inport
  Unit Delay : UnitDelay  InitialCondition=LANE_LINE_TRACK  SampleTime=-1
  TrackParamPred : Outport
  wires:
  TrackParamPrev/1 -> Unit Delay/1
  Unit Delay/1 -> TrackParamPred/1

== system Fusion_Frame_Model_Architecture/SENSOR_FUSION_SYSTEM/ROAD_GEOMETRY_CAMERA_FUSION/EGO_LANE_RIGHT_BOUNDARY_LINE_FUSION/LINE_TRACK_MANAGER ==
  UnGatedMeasIndex : Inport
  TrackParamUpd_in : Inport  Port=2
  Line_Measurements : Inport  Port=3
  Bus Creator : BusCreator  Inputs=7  OutDataTypeStr=Bus: ClothoidParamBus  NonVirtualBus=on
      settings: InheritFromInputs=off
  Bus Selector : BusSelector  OutputSignals=LateralOffset,HeadingAngle,Curvature,CurvatureDerivative,CurveLengthStart,CurveLength,ErrCOV
  Terminator : Terminator
  Terminator1 : Terminator
  TrackParamUpd : Outport
  wires:
  UnGatedMeasIndex/1 -> Terminator/1
  Line_Measurements/1 -> Terminator1/1
  Bus Selector/7 -> Bus Creator/7  "<ErrCOV>"
  Bus Selector/3 -> Bus Creator/3  "<Curvature>"
  Bus Creator/1 -> TrackParamUpd/1
  Bus Selector/4 -> Bus Creator/4  "<CurvatureDerivative>"
  Bus Selector/6 -> Bus Creator/6  "<CurveLength>"
  Bus Selector/1 -> Bus Creator/1  "<LateralOffset>"
  Bus Selector/2 -> Bus Creator/2  "<HeadingAngle>"
  Bus Selector/5 -> Bus Creator/5  "<CurveLengthStart>"
  TrackParamUpd_in/1 -> Bus Selector/1

== system Fusion_Frame_Model_Architecture/SENSOR_FUSION_SYSTEM/ROAD_GEOMETRY_CAMERA_FUSION/EGO_LANE_WIDTH_ESTIMATION/COMPUTE_SLOPE_AT_THE_POINTS ==
  SMALLER_CURVE : Inport
  POINTS : Inport  Port=2
  Ground : Ground
  Terminator : Terminator
  Terminator1 : Terminator
  SLOPE : Outport
  wires:
  SMALLER_CURVE/1 -> Terminator/1
  Ground/1 -> SLOPE/1
  POINTS/1 -> Terminator1/1

== system Fusion_Frame_Model_Architecture/SENSOR_FUSION_SYSTEM/ROAD_GEOMETRY_CAMERA_FUSION/EGO_LANE_WIDTH_ESTIMATION/COMPUTE_WIDTH_ALONG_THE_POINTS ==
  SLOPE : Inport
  POINTS_SMALLER_CURVE : Inport  Port=2
  POINTS_LARGER_CURVE : Inport  Port=3
  Terminator : Terminator
  Terminator1 : Terminator
  Terminator2 : Terminator
  WIDTH : Outport
  wires:
  POINTS_SMALLER_CURVE/1 -> Terminator/1
  ? -> WIDTH/1
  POINTS_LARGER_CURVE/1 -> Terminator1/1
  SLOPE/1 -> Terminator2/1

== system Fusion_Frame_Model_Architecture/SENSOR_FUSION_SYSTEM/ROAD_GEOMETRY_CAMERA_FUSION/EGO_LANE_WIDTH_ESTIMATION/ESTIMATE_EGO_LANE_WIDTH ==
  WIDTH_prev : Inport
  WIDTH_Measurements : Inport  Port=2
  Bus Creator : BusCreator  Inputs=2
  Bus Selector : BusSelector  OutputSignals=mean,variance
  Terminator : Terminator
  Unit Delay : UnitDelay  SampleTime=-1
  Unit Delay1 : UnitDelay  SampleTime=-1
  WIDTH_Upd : Outport
  wires:
  WIDTH_Measurements/1 -> Terminator/1
  Bus Selector/1 -> Unit Delay/1  "<mean>"
  Unit Delay1/1 -> Bus Creator/2  "variance"
  Bus Selector/2 -> Unit Delay1/1  "<variance>"
  Bus Creator/1 -> WIDTH_Upd/1
  WIDTH_prev/1 -> Bus Selector/1
  Unit Delay/1 -> Bus Creator/1  "mean"

== system Fusion_Frame_Model_Architecture/SENSOR_FUSION_SYSTEM/ROAD_GEOMETRY_CAMERA_FUSION/EGO_LANE_WIDTH_ESTIMATION/INTERPOLATE_POINTS_ON_SMALLER_CURVE ==
  SMALLER_CURVE : Inport
  Ground : Ground
  Terminator : Terminator
  POINTS : Outport
  wires:
  SMALLER_CURVE/1 -> Terminator/1
  Ground/1 -> POINTS/1

== system Fusion_Frame_Model_Architecture/SENSOR_FUSION_SYSTEM/ROAD_GEOMETRY_CAMERA_FUSION/EGO_LANE_WIDTH_ESTIMATION/LOCATE_POINTS_WITH_SAME_SLOPE ==
  SLOPE : Inport
  LARGER_CURVE : Inport  Port=2
  Ground : Ground
  Terminator : Terminator
  Terminator1 : Terminator
  POINTS : Outport
  wires:
  LARGER_CURVE/1 -> Terminator/1
  Ground/1 -> POINTS/1
  SLOPE/1 -> Terminator1/1

== system Fusion_Frame_Model_Architecture/SENSOR_FUSION_SYSTEM/ROAD_GEOMETRY_CAMERA_FUSION/EGO_LANE_WIDTH_ESTIMATION/SELECT_CURVE_WITH_SMALLER_LENGTH ==
  EGO_LANE_RIGHT_LINE_TRACK : Inport
  EGO_LANE_LEFT_LINE_TRACK : Inport  Port=2
  SMALLER_CURVE : Outport
  LARGER_CURVE : Outport  Port=2
  wires:
  EGO_LANE_RIGHT_LINE_TRACK/1 -> SMALLER_CURVE/1
  EGO_LANE_LEFT_LINE_TRACK/1 -> LARGER_CURVE/1

== system Fusion_Frame_Model_Architecture/SENSOR_FUSION_SYSTEM/ROAD_GEOMETRY_CAMERA_FUSION/ROAD_GEOMERY_AND_GRID_COMPUTATION/COMPUTE_LEFT_LINE ==
  OFFSET : Inport
  EGO_LANE_CENTER_LINE_TRACK : Inport  Port=2
  CURVE_FITTING_BY_LEAST_SQUARES : Subsystem
  GENERATE_POINTS_ON_THE_LANE_BORDER : Subsystem
  INTERPOLATE_POINTS_ALONG_THE_EGO_LANE_CENTER_LINE : Subsystem
  POLYNOMIAL_TO_CLOTHOID_CONVERSION : Subsystem
  L : Outport
  wires:
  EGO_LANE_CENTER_LINE_TRACK/1 -> INTERPOLATE_POINTS_ALONG_THE_EGO_LANE_CENTER_LINE/1(EGO_LANE_CENTER_LINE_TRACK)
  INTERPOLATE_POINTS_ALONG_THE_EGO_LANE_CENTER_LINE/1(PointsAlongTheLine) -> GENERATE_POINTS_ON_THE_LANE_BORDER/1(PointsAlongTheLine)
  OFFSET/1 -> GENERATE_POINTS_ON_THE_LANE_BORDER/2(EgoLaneWidth)
  GENERATE_POINTS_ON_THE_LANE_BORDER/1(PointsAlongTheLinea) -> CURVE_FITTING_BY_LEAST_SQUARES/1(Points)
  POLYNOMIAL_TO_CLOTHOID_CONVERSION/1(ClothoidCoefficients) -> L/1
  CURVE_FITTING_BY_LEAST_SQUARES/1(PolynomialCoefficients) -> POLYNOMIAL_TO_CLOTHOID_CONVERSION/1(PolynomialCoefficients)

== system Fusion_Frame_Model_Architecture/SENSOR_FUSION_SYSTEM/ROAD_GEOMETRY_CAMERA_FUSION/ROAD_GEOMERY_AND_GRID_COMPUTATION/COMPUTE_NEXT_LEFT_LINE ==
  OFFSET : Inport
  EGO_LANE_CENTER_LINE_TRACK : Inport  Port=2
  CURVE_FITTING_BY_LEAST_SQUARES : Subsystem
  GENERATE_POINTS_ON_THE_LANE_BORDER : Subsystem
  INTERPOLATE_POINTS_ALONG_THE_EGO_LANE_CENTER_LINE : Subsystem
  POLYNOMIAL_TO_CLOTHOID_CONVERSION : Subsystem
  NL : Outport
  wires:
  EGO_LANE_CENTER_LINE_TRACK/1 -> INTERPOLATE_POINTS_ALONG_THE_EGO_LANE_CENTER_LINE/1(EGO_LANE_CENTER_LINE_TRACK)
  INTERPOLATE_POINTS_ALONG_THE_EGO_LANE_CENTER_LINE/1(PointsAlongTheLine) -> GENERATE_POINTS_ON_THE_LANE_BORDER/1(PointsAlongTheLine)
  OFFSET/1 -> GENERATE_POINTS_ON_THE_LANE_BORDER/2(EgoLaneWidth)
  GENERATE_POINTS_ON_THE_LANE_BORDER/1(PointsAlongTheLinea) -> CURVE_FITTING_BY_LEAST_SQUARES/1(Points)
  POLYNOMIAL_TO_CLOTHOID_CONVERSION/1(ClothoidCoefficients) -> NL/1
  CURVE_FITTING_BY_LEAST_SQUARES/1(PolynomialCoefficients) -> POLYNOMIAL_TO_CLOTHOID_CONVERSION/1(PolynomialCoefficients)

== system Fusion_Frame_Model_Architecture/SENSOR_FUSION_SYSTEM/ROAD_GEOMETRY_CAMERA_FUSION/ROAD_GEOMERY_AND_GRID_COMPUTATION/COMPUTE_NEXT_NEXT_LEFT_LINE ==
  OFFSET : Inport
  EGO_LANE_CENTER_LINE_TRACK : Inport  Port=2
  CURVE_FITTING_BY_LEAST_SQUARES : Subsystem
  GENERATE_POINTS_ON_THE_LANE_BORDER : Subsystem
  INTERPOLATE_POINTS_ALONG_THE_EGO_LANE_CENTER_LINE : Subsystem
  POLYNOMIAL_TO_CLOTHOID_CONVERSION : Subsystem
  NNL : Outport
  wires:
  EGO_LANE_CENTER_LINE_TRACK/1 -> INTERPOLATE_POINTS_ALONG_THE_EGO_LANE_CENTER_LINE/1(EGO_LANE_CENTER_LINE_TRACK)
  INTERPOLATE_POINTS_ALONG_THE_EGO_LANE_CENTER_LINE/1(PointsAlongTheLine) -> GENERATE_POINTS_ON_THE_LANE_BORDER/1(PointsAlongTheLine)
  OFFSET/1 -> GENERATE_POINTS_ON_THE_LANE_BORDER/2(EgoLaneWidth)
  GENERATE_POINTS_ON_THE_LANE_BORDER/1(PointsAlongTheLinea) -> CURVE_FITTING_BY_LEAST_SQUARES/1(Points)
  POLYNOMIAL_TO_CLOTHOID_CONVERSION/1(ClothoidCoefficients) -> NNL/1
  CURVE_FITTING_BY_LEAST_SQUARES/1(PolynomialCoefficients) -> POLYNOMIAL_TO_CLOTHOID_CONVERSION/1(PolynomialCoefficients)

== system Fusion_Frame_Model_Architecture/SENSOR_FUSION_SYSTEM/ROAD_GEOMETRY_CAMERA_FUSION/ROAD_GEOMERY_AND_GRID_COMPUTATION/COMPUTE_NEXT_NEXT_RIGHT_LINE ==
  EGO_LANE_CENTER_LINE_TRACK : Inport
  OFFSET : Inport  Port=2
  CURVE_FITTING_BY_LEAST_SQUARES : Subsystem
  GENERATE_POINTS_ON_THE_LANE_BORDER : Subsystem
  INTERPOLATE_POINTS_ALONG_THE_EGO_LANE_CENTER_LINE : Subsystem
  POLYNOMIAL_TO_CLOTHOID_CONVERSION : Subsystem
  NNR : Outport
  wires:
  EGO_LANE_CENTER_LINE_TRACK/1 -> INTERPOLATE_POINTS_ALONG_THE_EGO_LANE_CENTER_LINE/1(EGO_LANE_CENTER_LINE_TRACK)
  INTERPOLATE_POINTS_ALONG_THE_EGO_LANE_CENTER_LINE/1(PointsAlongTheLine) -> GENERATE_POINTS_ON_THE_LANE_BORDER/1(PointsAlongTheLine)
  OFFSET/1 -> GENERATE_POINTS_ON_THE_LANE_BORDER/2(EgoLaneWidth)
  GENERATE_POINTS_ON_THE_LANE_BORDER/1(PointsAlongTheLinea) -> CURVE_FITTING_BY_LEAST_SQUARES/1(Points)
  POLYNOMIAL_TO_CLOTHOID_CONVERSION/1(ClothoidCoefficients) -> NNR/1
  CURVE_FITTING_BY_LEAST_SQUARES/1(PolynomialCoefficients) -> POLYNOMIAL_TO_CLOTHOID_CONVERSION/1(PolynomialCoefficients)

== system Fusion_Frame_Model_Architecture/SENSOR_FUSION_SYSTEM/ROAD_GEOMETRY_CAMERA_FUSION/ROAD_GEOMERY_AND_GRID_COMPUTATION/COMPUTE_NEXT_RIGHT_LINE ==
  EGO_LANE_CENTER_LINE_TRACK : Inport
  OFFSET : Inport  Port=2
  CURVE_FITTING_BY_LEAST_SQUARES : Subsystem
  GENERATE_POINTS_ON_THE_LANE_BORDER : Subsystem
  INTERPOLATE_POINTS_ALONG_THE_EGO_LANE_CENTER_LINE : Subsystem
  POLYNOMIAL_TO_CLOTHOID_CONVERSION : Subsystem
  NR : Outport
  wires:
  EGO_LANE_CENTER_LINE_TRACK/1 -> INTERPOLATE_POINTS_ALONG_THE_EGO_LANE_CENTER_LINE/1(EGO_LANE_CENTER_LINE_TRACK)
  INTERPOLATE_POINTS_ALONG_THE_EGO_LANE_CENTER_LINE/1(PointsAlongTheLine) -> GENERATE_POINTS_ON_THE_LANE_BORDER/1(PointsAlongTheLine)
  OFFSET/1 -> GENERATE_POINTS_ON_THE_LANE_BORDER/2(EgoLaneWidth)
  GENERATE_POINTS_ON_THE_LANE_BORDER/1(PointsAlongTheLinea) -> CURVE_FITTING_BY_LEAST_SQUARES/1(Points)
  POLYNOMIAL_TO_CLOTHOID_CONVERSION/1(ClothoidCoefficients) -> NR/1
  CURVE_FITTING_BY_LEAST_SQUARES/1(PolynomialCoefficients) -> POLYNOMIAL_TO_CLOTHOID_CONVERSION/1(PolynomialCoefficients)

== system Fusion_Frame_Model_Architecture/SENSOR_FUSION_SYSTEM/ROAD_GEOMETRY_CAMERA_FUSION/ROAD_GEOMERY_AND_GRID_COMPUTATION/COMPUTE_OFFSET ==
  Width : Inport
  Bus Selector : BusSelector  OutputSignals=mean
  Offset : Outport
  wires:
  Width/1 -> Bus Selector/1
  Bus Selector/1 -> Offset/1  "<mean>"

== system Fusion_Frame_Model_Architecture/SENSOR_FUSION_SYSTEM/ROAD_GEOMETRY_CAMERA_FUSION/ROAD_GEOMERY_AND_GRID_COMPUTATION/COMPUTE_OFFSET1 ==
  Width : Inport
  Bus Selector : BusSelector  OutputSignals=mean
  Offset : Outport
  wires:
  Width/1 -> Bus Selector/1
  Bus Selector/1 -> Offset/1  "<mean>"

== system Fusion_Frame_Model_Architecture/SENSOR_FUSION_SYSTEM/ROAD_GEOMETRY_CAMERA_FUSION/ROAD_GEOMERY_AND_GRID_COMPUTATION/COMPUTE_OFFSET2 ==
  Width : Inport
  Bus Selector : BusSelector  OutputSignals=mean
  Offset : Outport
  wires:
  Width/1 -> Bus Selector/1
  Bus Selector/1 -> Offset/1  "<mean>"

== system Fusion_Frame_Model_Architecture/SENSOR_FUSION_SYSTEM/ROAD_GEOMETRY_CAMERA_FUSION/ROAD_GEOMERY_AND_GRID_COMPUTATION/COMPUTE_OFFSET3 ==
  Width : Inport
  Bus Selector : BusSelector  OutputSignals=mean
  Offset : Outport
  wires:
  Width/1 -> Bus Selector/1
  Bus Selector/1 -> Offset/1  "<mean>"

== system Fusion_Frame_Model_Architecture/SENSOR_FUSION_SYSTEM/ROAD_GEOMETRY_CAMERA_FUSION/ROAD_GEOMERY_AND_GRID_COMPUTATION/COMPUTE_OFFSET4 ==
  Width : Inport
  Bus Selector : BusSelector  OutputSignals=mean
  Offset : Outport
  wires:
  Width/1 -> Bus Selector/1
  Bus Selector/1 -> Offset/1  "<mean>"

== system Fusion_Frame_Model_Architecture/SENSOR_FUSION_SYSTEM/ROAD_GEOMETRY_CAMERA_FUSION/ROAD_GEOMERY_AND_GRID_COMPUTATION/COMPUTE_OFFSET5 ==
  Width : Inport
  Bus Selector : BusSelector  OutputSignals=mean
  Offset : Outport
  wires:
  Width/1 -> Bus Selector/1
  Bus Selector/1 -> Offset/1  "<mean>"

== system Fusion_Frame_Model_Architecture/SENSOR_FUSION_SYSTEM/ROAD_GEOMETRY_CAMERA_FUSION/ROAD_GEOMERY_AND_GRID_COMPUTATION/COMPUTE_RIGHT_LINE ==
  EGO_LANE_CENTER_LINE_TRACK : Inport
  OFFSET : Inport  Port=2
  CURVE_FITTING_BY_LEAST_SQUARES : Subsystem
  GENERATE_POINTS_ON_THE_LANE_BORDER : Subsystem
  INTERPOLATE_POINTS_ALONG_THE_EGO_LANE_CENTER_LINE : Subsystem
  POLYNOMIAL_TO_CLOTHOID_CONVERSION : Subsystem
  R : Outport
  wires:
  EGO_LANE_CENTER_LINE_TRACK/1 -> INTERPOLATE_POINTS_ALONG_THE_EGO_LANE_CENTER_LINE/1(EGO_LANE_CENTER_LINE_TRACK)
  INTERPOLATE_POINTS_ALONG_THE_EGO_LANE_CENTER_LINE/1(PointsAlongTheLine) -> GENERATE_POINTS_ON_THE_LANE_BORDER/1(PointsAlongTheLine)
  OFFSET/1 -> GENERATE_POINTS_ON_THE_LANE_BORDER/2(EgoLaneWidth)
  GENERATE_POINTS_ON_THE_LANE_BORDER/1(PointsAlongTheLinea) -> CURVE_FITTING_BY_LEAST_SQUARES/1(Points)
  POLYNOMIAL_TO_CLOTHOID_CONVERSION/1(ClothoidCoefficients) -> R/1
  CURVE_FITTING_BY_LEAST_SQUARES/1(PolynomialCoefficients) -> POLYNOMIAL_TO_CLOTHOID_CONVERSION/1(PolynomialCoefficients)

== system Fusion_Frame_Model_Architecture/SENSOR_FUSION_SYSTEM/ROAD_GEOMETRY_CAMERA_FUSION/ROAD_GEOMERY_AND_GRID_COMPUTATION/COMPUTE_ROAD_GRID ==
  RoadGeometry : Inport
  EGO_Param : Inport  Port=2
  GRID_Prev : Inport  Port=3
  DISTANCE_TRAVELLED_BY_EGO_VEHICLE_DURING_DT : Subsystem
  EGO_COMPENSATION_FOR_ROAD_GRID_PREDICTION : Subsystem
  ROAD_GRID_UPDATE : Subsystem
  GRID_Upd : Outport
  wires:
  GRID_Prev/1 -> EGO_COMPENSATION_FOR_ROAD_GRID_PREDICTION/1(ROAD_GRID_prev)
  EGO_Param/1 -> DISTANCE_TRAVELLED_BY_EGO_VEHICLE_DURING_DT/1(EgoParam)
  RoadGeometry/1 -> ROAD_GRID_UPDATE/2(RPAD_GEOMETRY)
  DISTANCE_TRAVELLED_BY_EGO_VEHICLE_DURING_DT/1(dYaw) -> EGO_COMPENSATION_FOR_ROAD_GRID_PREDICTION/2(dYaw)
  DISTANCE_TRAVELLED_BY_EGO_VEHICLE_DURING_DT/2(dX) -> EGO_COMPENSATION_FOR_ROAD_GRID_PREDICTION/3(dX)
  DISTANCE_TRAVELLED_BY_EGO_VEHICLE_DURING_DT/3(dY) -> EGO_COMPENSATION_FOR_ROAD_GRID_PREDICTION/4(dY)
  EGO_COMPENSATION_FOR_ROAD_GRID_PREDICTION/1(ROAD_GRID_egoCompensated) -> ROAD_GRID_UPDATE/1(ROAD_GRID_Pred)
  ROAD_GRID_UPDATE/1(ROAD_GRID_Upd) -> GRID_Upd/1

== system Fusion_Frame_Model_Architecture/SENSOR_FUSION_SYSTEM/ROAD_GEOMETRY_CAMERA_FUSION/ROAD_GEOMERY_AND_GRID_COMPUTATION/SET_DATA ==
  EGO_LANE_NEXT_NEXT_LEFT_BOUNDARY : Inport
  EGO_LANE_NEXT_LEFT_BOUNDARY : Inport  Port=2
  EGO_LANE_LEFT_BOUNDARY : Inport  Port=3
  EGO_LANE_CENTER_TRACK_ESTIMATION : Inport  Port=4
  EGO_LANE_RIGHT_BOUNDARY : Inport  Port=5
  EGO_LANE_NEXT_RIGHT_BOUNDARY : Inport  Port=6
  EGO_LANE_NEXT_NEXT_RIGHT_BOUNDARY : Inport  Port=7
  Bus Creator : BusCreator  Inputs=7  OutDataTypeStr=Bus: ROAD_GEOMETRY  NonVirtualBus=on
      settings: InheritFromInputs=off
  ROAD : Outport
  wires:
  EGO_LANE_LEFT_BOUNDARY/1 -> Bus Creator/3
  EGO_LANE_NEXT_NEXT_RIGHT_BOUNDARY/1 -> Bus Creator/7
  EGO_LANE_NEXT_LEFT_BOUNDARY/1 -> Bus Creator/2
  EGO_LANE_NEXT_NEXT_LEFT_BOUNDARY/1 -> Bus Creator/1
  Bus Creator/1 -> ROAD/1
  EGO_LANE_CENTER_TRACK_ESTIMATION/1 -> Bus Creator/4
  EGO_LANE_NEXT_RIGHT_BOUNDARY/1 -> Bus Creator/6
  EGO_LANE_RIGHT_BOUNDARY/1 -> Bus Creator/5

== system Fusion_Frame_Model_Architecture/SENSOR_FUSION_SYSTEM/ROAD_GEOMETRY_CAMERA_FUSION/SPATIAL_ALLIGNMENT_CLOTHOID_COEFFICIENTS/CLUSTER_LINE_MEASUREMENTS ==
  EGO_LANE_BOUNDARY_LINE_MEAS : Inport
  LINE_CLUSTERS : Outport
  wires:
  EGO_LANE_BOUNDARY_LINE_MEAS/1 -> LINE_CLUSTERS/1

== system Fusion_Frame_Model_Architecture/SENSOR_FUSION_SYSTEM/ROAD_GEOMETRY_CAMERA_FUSION/SPATIAL_ALLIGNMENT_CLOTHOID_COEFFICIENTS/SEGREGATE_LINE_MEASUREMENTS_AS_LEFT_AND_RIGHT_MEASUREMENTS ==
  EGO_LANE_BOUNDARY_LINE_MEAS : Inport
  LINE_CLUSTERS : Inport  Port=2
  Terminator : Terminator
  EGO_LANE_LEFT_BOUNDARY_LINE_MEAS : Outport
  EGO_LANE_RIGHT_BOUNDARY_LINE_MEAS : Outport  Port=2
  wires:
  EGO_LANE_BOUNDARY_LINE_MEAS/1 -> EGO_LANE_RIGHT_BOUNDARY_LINE_MEAS/1, EGO_LANE_LEFT_BOUNDARY_LINE_MEAS/1
  LINE_CLUSTERS/1 -> Terminator/1

== system Fusion_Frame_Model_Architecture/SENSOR_FUSION_SYSTEM/ROAD_GEOMETRY_CAMERA_FUSION/SPATIAL_ALLIGNMENT_CLOTHOID_COEFFICIENTS/SPATIAL_ALLIGNMENT_LINE_CLOTHOID_MEASUREMENTS ==
  CAM_SENSOR_PARAM : Inport
  LINE_CLOTHOID_MEASUREMENTS : Inport  Port=2
  Bus Creator : BusCreator  Inputs=5  OutDataTypeStr=Bus: LINE_MEAS_MAT_CTS  NonVirtualBus=on
      settings: InheritFromInputs=off
  Constant : Constant  Value=single(zeros(5, 100))
  Constant1 : Constant  Value=single(zeros(5, 5, 100))
  Constant2 : Constant  Value=uint16(zeros(2, 100))
  Constant3 : Constant  Value=uint16(zeros(1, 8))
  Constant4 : Constant  Value=uint16(zeros(1, 8))
  Terminator : Terminator
  Terminator1 : Terminator
  EGO_LANE_BOUNDARY_LINE_MEAS : Outport
  wires:
  CAM_SENSOR_PARAM/1 -> Terminator/1
  LINE_CLOTHOID_MEASUREMENTS/1 -> Terminator1/1
  Constant/1 -> Bus Creator/1  "MeasArray"
  Constant1/1 -> Bus Creator/2  "MeasCovariance"
  Constant2/1 -> Bus Creator/3  "MeasRef"
  Constant3/1 -> Bus Creator/4  "ValidMeasCount"
  Constant4/1 -> Bus Creator/5  "ValidCumulativeMeasCount"
  Bus Creator/1 -> EGO_LANE_BOUNDARY_LINE_MEAS/1

== system Fusion_Frame_Model_Architecture/SENSOR_FUSION_SYSTEM/ROAD_GEOMETRY_CAMERA_FUSION/SPATIAL_ALLIGNMENT_CLOTHOID_COEFFICIENTS/TEMPORAL_ALLIGNMENT_LINE_CLOTHOID_MEASUREMENTS ==
  EGO_LANE_BOUNDARY_LINE_MEAS_in : Inport
  EGO_LANE_BOUNDARY_LINE_MEAS : Outport
  wires:
  EGO_LANE_BOUNDARY_LINE_MEAS_in/1 -> EGO_LANE_BOUNDARY_LINE_MEAS/1

== system Fusion_Frame_Model_Architecture/SENSOR_MEASUREMENTS/RADAR_CAMERA_EGO_SENSOR_INTERFACE/CameraSensors/Camera1 ==
  timeIdx : Inport
  nObjCamera : Inport  Port=2
  SensorMeas : Inport  Port=3
  CHECK_IF_DATA_IS_VALID : Subsystem
  GET_DATA : Subsystem
  LOOP_OVER_CAMERAS : ForIterator  ResetStates=reset  IterationSource=external  IterationVariableDataType=int16
  SET_DATA : Subsystem
  Selector : Selector  InputPortWidth=nCameras  IndexOptions=Index vector (dialog)  Indices=1  OutputSizes=1
  C1 : Outport
  wires:
  nObjCamera/1 -> Selector/1
  LOOP_OVER_CAMERAS/1 -> [index]
  GET_DATA/5(OBJ_TYPE) -> SET_DATA/7(OBJ_TYPE)
  [px] -> SET_DATA/2(px)  "px"
  GET_DATA/7(measCaptureTime) -> SET_DATA/9(TIME_STAMP)
  SET_DATA/1(C1) -> C1/1
  [vx] -> SET_DATA/4(vx)  "vx"
  GET_DATA/1(PX) -> CHECK_IF_DATA_IS_VALID/2(px), [px]
  Selector/1 -> LOOP_OVER_CAMERAS/1
  GET_DATA/3(VX) -> CHECK_IF_DATA_IS_VALID/4(vx), [vx]
  timeIdx/1 -> GET_DATA/2(time)
  CHECK_IF_DATA_IS_VALID/1(ID) -> SET_DATA/6(id)
  SensorMeas/1 -> SET_DATA/1(SensorData)
  GET_DATA/6(NOISE_COV) -> SET_DATA/8(NOISE_COV)
  [vy] -> SET_DATA/5(vy)  "vy"
  [py] -> SET_DATA/3(py)  "py"
  GET_DATA/4(VY) -> CHECK_IF_DATA_IS_VALID/5(vy), [vy]
  GET_DATA/2(PY) -> CHECK_IF_DATA_IS_VALID/3(py), [py]
  [index] -> SET_DATA/10(iter), CHECK_IF_DATA_IS_VALID/1(idx), GET_DATA/1(idx)

== system Fusion_Frame_Model_Architecture/SENSOR_MEASUREMENTS/RADAR_CAMERA_EGO_SENSOR_INTERFACE/CameraSensors/Camera2 ==
  timeIdx : Inport
  nObjCamera : Inport  Port=2
  SensorMeas : Inport  Port=3
  ExtractMeasParam1 : Subsystem
  For Iterator : ForIterator  ResetStates=reset  IterationSource=external  IterationVariableDataType=int16
  IsValid2 : Subsystem
  Selector : Selector  InputPortWidth=nCameras  IndexOptions=Starting index (dialog)  Indices=2  OutputSizes=1
  Subsystem1 : Subsystem
  C2 : Outport
  wires:
  ExtractMeasParam1/1(PX) -> IsValid2/2(px), [px]
  ExtractMeasParam1/7(measCaptureTime) -> Subsystem1/9(TIME_STAMP)
  IsValid2/1(ID) -> Subsystem1/6(id)
  [vy] -> Subsystem1/5(vy)  "vy"
  ExtractMeasParam1/6(NOISE_COV) -> Subsystem1/8(NOISE_COV)
  [vx] -> Subsystem1/4(vx)  "vx"
  SensorMeas/1 -> Subsystem1/1(SensorData)
  nObjCamera/1 -> Selector/1
  [py] -> Subsystem1/3(py)  "py"
  For Iterator/1 -> [index]
  [index] -> Subsystem1/10(iter), IsValid2/1(idx), ExtractMeasParam1/1(idx)
  ExtractMeasParam1/4(VY) -> IsValid2/5(vy), [vy]
  [px] -> Subsystem1/2(px)  "px"
  Selector/1 -> For Iterator/1
  ExtractMeasParam1/2(PY) -> IsValid2/3(py), [py]
  Subsystem1/1(C2) -> C2/1
  ExtractMeasParam1/5(OBJ_TYPE) -> Subsystem1/7(OBJ_TYPE)
  timeIdx/1 -> ExtractMeasParam1/2(time)
  ExtractMeasParam1/3(VX) -> IsValid2/4(vx), [vx]

== system Fusion_Frame_Model_Architecture/SENSOR_MEASUREMENTS/RADAR_CAMERA_EGO_SENSOR_INTERFACE/CameraSensors/Camera3 ==
  timeIdx : Inport
  nObjCamera : Inport  Port=2
  SensorMeas : Inport  Port=3
  ExtractMeasParam1 : Subsystem
  For Iterator : ForIterator  ResetStates=reset  IterationSource=external  IterationVariableDataType=int16
  IsValid2 : Subsystem
  Selector : Selector  InputPortWidth=nCameras  IndexOptions=Starting index (dialog)  Indices=3  OutputSizes=1
  Subsystem1 : Subsystem
  C3 : Outport
  wires:
  ExtractMeasParam1/1(PX) -> IsValid2/2(px), [px]
  ExtractMeasParam1/7(measCaptureTime) -> Subsystem1/9(TIME_STAMP)
  IsValid2/1(ID) -> Subsystem1/6(id)
  [vy] -> Subsystem1/5(vy)  "vy"
  ExtractMeasParam1/6(NOISE_COV) -> Subsystem1/8(NOISE_COV)
  [vx] -> Subsystem1/4(vx)  "vx"
  SensorMeas/1 -> Subsystem1/1(SensorData)
  nObjCamera/1 -> Selector/1
  [py] -> Subsystem1/3(py)  "py"
  For Iterator/1 -> [index]
  [index] -> Subsystem1/10(iter), IsValid2/1(idx), ExtractMeasParam1/1(idx)
  ExtractMeasParam1/4(VY) -> IsValid2/5(vy), [vy]
  [px] -> Subsystem1/2(px)  "px"
  Selector/1 -> For Iterator/1
  ExtractMeasParam1/2(PY) -> IsValid2/3(py), [py]
  Subsystem1/1(C3) -> C3/1
  ExtractMeasParam1/5(OBJ_TYPE) -> Subsystem1/7(OBJ_TYPE)
  timeIdx/1 -> ExtractMeasParam1/2(time)
  ExtractMeasParam1/3(VX) -> IsValid2/4(vx), [vx]

== system Fusion_Frame_Model_Architecture/SENSOR_MEASUREMENTS/RADAR_CAMERA_EGO_SENSOR_INTERFACE/CameraSensors/Camera4 ==
  timeIdx : Inport
  nObjCamera : Inport  Port=2
  SensorMeas : Inport  Port=3
  ExtractMeasParam1 : Subsystem
  For Iterator : ForIterator  ResetStates=reset  IterationSource=external  IterationVariableDataType=int16
  IsValid2 : Subsystem
  Selector : Selector  InputPortWidth=nCameras  IndexOptions=Starting index (dialog)  Indices=4  OutputSizes=1
  Subsystem1 : Subsystem
  C4 : Outport
  wires:
  ExtractMeasParam1/1(PX) -> IsValid2/2(px), [px]
  ExtractMeasParam1/7(measCaptureTime) -> Subsystem1/9(TIME_STAMP)
  IsValid2/1(ID) -> Subsystem1/6(id)
  [vy] -> Subsystem1/5(vy)  "vy"
  ExtractMeasParam1/6(NOISE_COV) -> Subsystem1/8(NOISE_COV)
  [vx] -> Subsystem1/4(vx)  "vx"
  SensorMeas/1 -> Subsystem1/1(SensorData)
  nObjCamera/1 -> Selector/1
  [py] -> Subsystem1/3(py)  "py"
  For Iterator/1 -> [index]
  [index] -> Subsystem1/10(iter), IsValid2/1(idx), ExtractMeasParam1/1(idx)
  ExtractMeasParam1/4(VY) -> IsValid2/5(vy), [vy]
  [px] -> Subsystem1/2(px)  "px"
  Selector/1 -> For Iterator/1
  ExtractMeasParam1/2(PY) -> IsValid2/3(py), [py]
  Subsystem1/1(C4) -> C4/1
  ExtractMeasParam1/5(OBJ_TYPE) -> Subsystem1/7(OBJ_TYPE)
  timeIdx/1 -> ExtractMeasParam1/2(time)
  ExtractMeasParam1/3(VX) -> IsValid2/4(vx), [vx]

== system Fusion_Frame_Model_Architecture/SENSOR_MEASUREMENTS/RADAR_CAMERA_EGO_SENSOR_INTERFACE/CameraSensors/Camera5 ==
  timeIdx : Inport
  nObjCamera : Inport  Port=2
  SensorMeas : Inport  Port=3
  ExtractMeasParam1 : Subsystem
  For Iterator : ForIterator  ResetStates=reset  IterationSource=external  IterationVariableDataType=int16
  IsValid2 : Subsystem
  Selector : Selector  InputPortWidth=nCameras  IndexOptions=Starting index (dialog)  Indices=5  OutputSizes=1
  Subsystem1 : Subsystem
  C5 : Outport
  wires:
  ExtractMeasParam1/1(PX) -> IsValid2/2(px), [px]
  ExtractMeasParam1/7(measCaptureTime) -> Subsystem1/9(TIME_STAMP)
  IsValid2/1(ID) -> Subsystem1/6(id)
  [vy] -> Subsystem1/5(vy)  "vy"
  ExtractMeasParam1/6(NOISE_COV) -> Subsystem1/8(NOISE_COV)
  [vx] -> Subsystem1/4(vx)  "vx"
  SensorMeas/1 -> Subsystem1/1(SensorData)
  nObjCamera/1 -> Selector/1
  [py] -> Subsystem1/3(py)  "py"
  For Iterator/1 -> [index]
  [index] -> Subsystem1/10(iter), IsValid2/1(idx), ExtractMeasParam1/1(idx)
  ExtractMeasParam1/4(VY) -> IsValid2/5(vy), [vy]
  [px] -> Subsystem1/2(px)  "px"
  Selector/1 -> For Iterator/1
  ExtractMeasParam1/2(PY) -> IsValid2/3(py), [py]
  Subsystem1/1(C5) -> C5/1
  ExtractMeasParam1/5(OBJ_TYPE) -> Subsystem1/7(OBJ_TYPE)
  timeIdx/1 -> ExtractMeasParam1/2(time)
  ExtractMeasParam1/3(VX) -> IsValid2/4(vx), [vx]

== system Fusion_Frame_Model_Architecture/SENSOR_MEASUREMENTS/RADAR_CAMERA_EGO_SENSOR_INTERFACE/CameraSensors/Camera6 ==
  timeIdx : Inport
  nObjCamera : Inport  Port=2
  SensorMeas : Inport  Port=3
  ExtractMeasParam1 : Subsystem
  For Iterator : ForIterator  ResetStates=reset  IterationSource=external  IterationVariableDataType=int16
  IsValid2 : Subsystem
  Selector : Selector  InputPortWidth=nCameras  IndexOptions=Starting index (dialog)  Indices=6  OutputSizes=1
  Subsystem1 : Subsystem
  C6 : Outport
  wires:
  ExtractMeasParam1/1(PX) -> IsValid2/2(px), [px]
  ExtractMeasParam1/7(measCaptureTime) -> Subsystem1/9(TIME_STAMP)
  IsValid2/1(ID) -> Subsystem1/6(id)
  [vy] -> Subsystem1/5(vy)  "vy"
  ExtractMeasParam1/6(NOISE_COV) -> Subsystem1/8(NOISE_COV)
  [vx] -> Subsystem1/4(vx)  "vx"
  SensorMeas/1 -> Subsystem1/1(SensorData)
  nObjCamera/1 -> Selector/1
  [py] -> Subsystem1/3(py)  "py"
  For Iterator/1 -> [index]
  [index] -> Subsystem1/10(iter), IsValid2/1(idx), ExtractMeasParam1/1(idx)
  ExtractMeasParam1/4(VY) -> IsValid2/5(vy), [vy]
  [px] -> Subsystem1/2(px)  "px"
  Selector/1 -> For Iterator/1
  ExtractMeasParam1/2(PY) -> IsValid2/3(py), [py]
  Subsystem1/1(C6) -> C6/1
  ExtractMeasParam1/5(OBJ_TYPE) -> Subsystem1/7(OBJ_TYPE)
  timeIdx/1 -> ExtractMeasParam1/2(time)
  ExtractMeasParam1/3(VX) -> IsValid2/4(vx), [vx]
